simulink model "GreenCraneLagrangian"  (R2020b)
settings: Solver=FixedStepAuto  StartTime=0.0  StopTime=20  FixedStep=0.001  RelTol=1e-3  EnableMultiTasking=on
settings Model: Creator=dpadova  LastModifiedBy=hagen
settings SolverCC: AlgebraicLoopSolver=LineSearch
settings DataIOCC: LimitDataPoints=on  SaveFormat=Array  ReturnWorkspaceOutputs=off
settings OptimizationCC: ExpressionDepthLimit=2147483647  EfficientMapNaN2IntZero=off  LifeSpan=inf
settings DebuggingCC: AlgebraicLoopMsg=none  UnderspecifiedInitializationDetection=Classic  MergeDetectMultiDrivingBlocksExec=none  MaxConsecutiveZCsMsg=warning  StateNameClashWarn=warning  SFUnexpectedBacktrackingDiag=warning  SFNoUnconditionalDefaultTransitionDiag=warning  SFExecutionAtInitializationDiag=none  ArithmeticOperatorsInVariantConditions=warning
settings HardwareCC: ProdBitPerPointer=32  ProdBitPerSizeT=32  ProdBitPerPtrDiffT=32  ProdLargestAtomicFloat=None  ProdIntDivRoundTo=Undefined  ProdEndianess=Unspecified  ProdWordSize=32  ProdHWDeviceType=32-bit Generic  TargetBitPerPointer=64  TargetBitPerSizeT=64  TargetBitPerPtrDiffT=64  TargetLongLongMode=on  TargetIntDivRoundTo=Zero  TargetEndianess=LittleEndian  TargetWordSize=64  TargetHWDeviceType=MATLAB Host  ProdEqTarget=off
settings ModelReferenceCC: PropagateSignalLabelsOutOfModel=off
settings SFSimCC: SimUseLocalCustomCode=off  CustomCodeUndefinedFunction=UseInterfaceOnly
settings RTWCC: RTWUseLocalCustomCode=off
settings CodeAppCC: MaxIdLength=128
settings GRTTargetCC: TargetLangStandard=C89/C90 (ANSI)  CombineOutputUpdateFcns=off  GRTInterface=on
settings ConfigComp: CovMetricSettings=dw  CovSaveCumulativeToWorkspaceVar=on  CovSaveSingleToWorkspaceVar=on  CovExternalEMLEnable=off

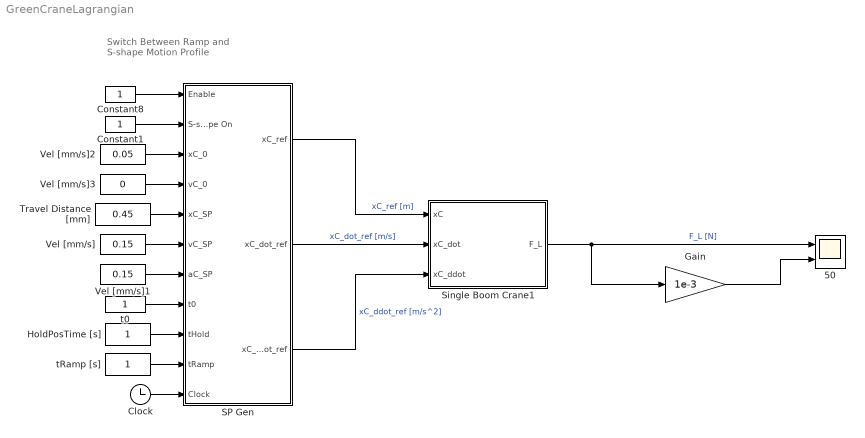
== system GreenCraneLagrangian ==
  note: Switch Between
      | Ramp and S-shape
      | Motion Profile
  50 : Scope  NumInputPorts=2
  Clock : Clock
  Constant1 : Constant  OutDataTypeStr=boolean
  Constant8 : Constant  OutDataTypeStr=boolean
  Gain : Gain  Gain=1e-3
  HoldPosTime [s] : Constant
  SP Gen : Subsystem
  Single Boom Crane1 : Subsystem
  Travel Distance [mm] : Constant  Value=0.45
  Vel [mm/s] : Constant  Value=0.15
  Vel [mm/s]1 : Constant  Value=0.15
  Vel [mm/s]2 : Constant  Value=0.05
  Vel [mm/s]3 : Constant  Value=0
  t0 : Constant
  tRamp [s] : Constant
  wires:
  Vel [mm/s]3/1 -> SP Gen/4(vC_0)
  t0/1 -> SP Gen/8(t0)
  HoldPosTime [s]/1 -> SP Gen/9(tHold)
  Clock/1 -> SP Gen/11(Clock)
  Travel Distance [mm]/1 -> SP Gen/5(xC_SP)
  Vel [mm/s]2/1 -> SP Gen/3(xC_0)
  Constant8/1 -> SP Gen/1(Enable)
  Vel [mm/s]/1 -> SP Gen/6(vC_SP)
  tRamp [s]/1 -> SP Gen/10(tRamp)
  Vel [mm/s]1/1 -> SP Gen/7(aC_SP)
  Constant1/1 -> SP Gen/2(S-shape On)
  SP Gen/1(xC_ref) -> Single Boom Crane1/1(xC)  "xC_ref [m]"
  SP Gen/2(xC_dot_ref) -> Single Boom Crane1/2(xC_dot)  "xC_dot_ref [m/s]"
  SP Gen/3("xC_ddot_ref ") -> Single Boom Crane1/3("xC_ddot ")  "xC_ddot_ref [m/s^2]"
  Single Boom Crane1/1(F_L) -> 50/1, Gain/1  "F_L [N]"
  Gain/1 -> 50/2

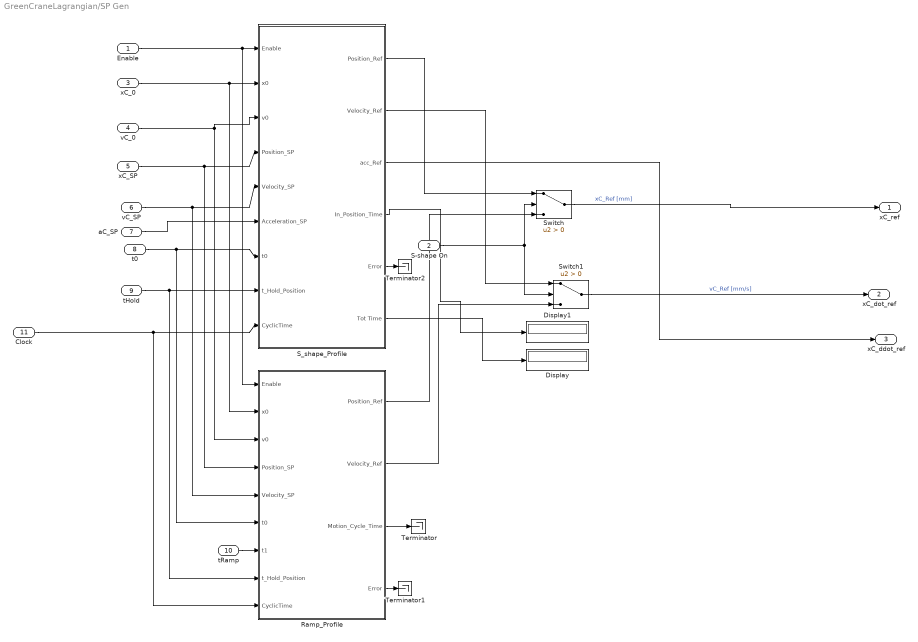
== system GreenCraneLagrangian/SP Gen ==
  Enable : Inport
  S-shape On : Inport  Port=2
  xC_0 : Inport  Port=3
  vC_0 : Inport  Port=4
  xC_SP : Inport  Port=5
  vC_SP : Inport  Port=6
  aC_SP : Inport  Port=7
  t0 : Inport  Port=8
  tHold : Inport  Port=9
  tRamp : Inport  Port=10
  Clock : Inport  Port=11
  Display : Display
  Display1 : Display
  Ramp_Profile : Subsystem  TreatAsAtomicUnit=on  VariantControl=Ramp_Profile
  S_shape_Profile : Subsystem  VariantControl=S_shape_Profile
  Switch : Switch  Criteria=u2 > Threshold
  Switch1 : Switch  Criteria=u2 > Threshold
  Terminator : Terminator
  Terminator1 : Terminator
  Terminator2 : Terminator
  xC_ref : Outport  VectorParamsAs1DForOutWhenUnconnected=off
  xC_dot_ref : Outport  Port=2  VectorParamsAs1DForOutWhenUnconnected=off
  "xC_ddot_ref " : Outport  Port=3  VectorParamsAs1DForOutWhenUnconnected=off
  wires:
  t0/1 -> Ramp_Profile/6(t0), S_shape_Profile/7(t0)
  vC_SP/1 -> Ramp_Profile/5(Velocity_SP), S_shape_Profile/5(Velocity_SP)
  xC_0/1 -> Ramp_Profile/2(x0), S_shape_Profile/2(x0)
  xC_SP/1 -> Ramp_Profile/4(Position_SP), S_shape_Profile/4(Position_SP)
  Enable/1 -> Ramp_Profile/1(Enable), S_shape_Profile/1(Enable)
  tHold/1 -> Ramp_Profile/8(t_Hold_Position), S_shape_Profile/8(t_Hold_Position)
  S_shape_Profile/1(Position_Ref) -> Switch/1
  Ramp_Profile/1(Position_Ref) -> Switch/3
  S_shape_Profile/2(Velocity_Ref) -> Switch1/1
  S-shape On/1 -> Switch/2, Switch1/2
  Ramp_Profile/2(Velocity_Ref) -> Switch1/3
  tRamp/1 -> Ramp_Profile/7(t1)
  S_shape_Profile/6(Tot Time) -> Display/1
  S_shape_Profile/4(" In_Position_Time") -> Display1/1
  vC_0/1 -> S_shape_Profile/3(v0), Ramp_Profile/3(v0)
  aC_SP/1 -> S_shape_Profile/6(Acceleration_SP)
  Clock/1 -> Ramp_Profile/9(CyclicTime), S_shape_Profile/9(CyclicTime)
  Switch/1 -> xC_ref/1  "xC_Ref [mm]"
  Switch1/1 -> xC_dot_ref/1  "vC_Ref [mm/s]"
  S_shape_Profile/3(acc_Ref) -> "xC_ddot_ref "/1
  Ramp_Profile/3(Motion_Cycle_Time) -> Terminator/1
  Ramp_Profile/4(Error) -> Terminator1/1
  S_shape_Profile/5(Error) -> Terminator2/1

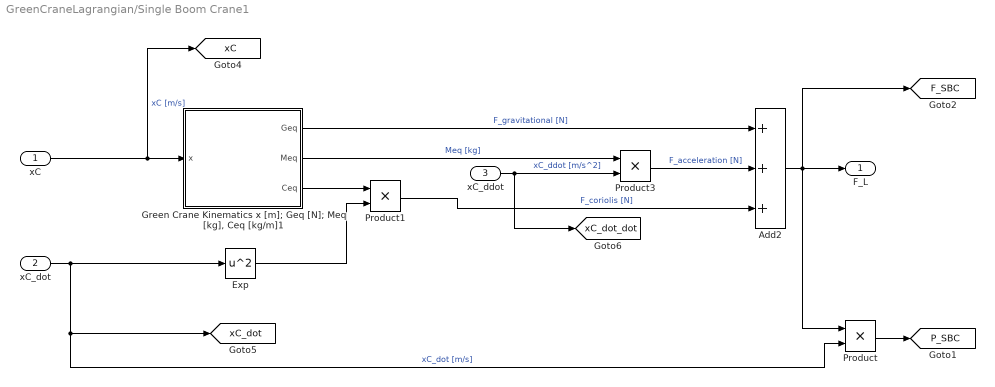
== system GreenCraneLagrangian/Single Boom Crane1 ==
  xC : Inport
  xC_dot : Inport  Port=2
  "xC_ddot " : Inport  Port=3
  Add2 : Sum  Inputs=+++
  Exp : Math  Operator=square  SaturateOnIntegerOverflow=on
  "Green Crane Kinematics x [m]; Geq [N]; Meq [kg], Ceq [kg/m]1" : MATLAB Function  TreatAsAtomicUnit=on
  Product : Product
  Product1 : Product
  Product3 : Product
  F_L : Outport
  tag scope: F_SBC=global, P_SBC=global, xC=global, xC_dot=global, xC_dot_dot=global
  wires:
  "Green Crane Kinematics x [m]; Geq [N]; Meq [kg], Ceq [kg/m]1"/2(Meq) -> Product3/1  "Meq [kg]"
  Add2/1 -> [F_SBC], Product/1, F_L/1
  "Green Crane Kinematics x [m]; Geq [N]; Meq [kg], Ceq [kg/m]1"/1(Geq) -> Add2/1  "F_gravitational [N]"
  Product3/1 -> Add2/2  "F_acceleration [N]"
  "Green Crane Kinematics x [m]; Geq [N]; Meq [kg], Ceq [kg/m]1"/3(Ceq) -> Product1/1
  Exp/1 -> Product1/2
  Product1/1 -> Add2/3  "F_coriolis [N]"
  "xC_ddot "/1 -> [xC_dot_dot], Product3/2  "xC_ddot [m/s^2]"
  xC_dot/1 -> Product/2, [xC_dot], Exp/1  "xC_dot [m/s]"
  xC/1 -> [xC], "Green Crane Kinematics x [m]; Geq [N]; Meq [kg], Ceq [kg/m]1"/1(x)  "xC [m/s]"
  Product/1 -> [P_SBC]

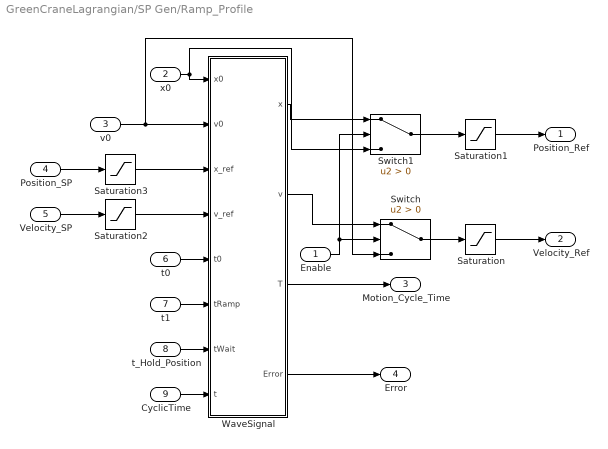
== system GreenCraneLagrangian/SP Gen/Ramp_Profile ==
  Enable : Inport  OutDataTypeStr=boolean
  x0 : Inport  Port=2
  v0 : Inport  Port=3
  Position_SP : Inport  Port=4
  Velocity_SP : Inport  Port=5
  t0 : Inport  Port=6
  t1 : Inport  Port=7
  t_Hold_Position : Inport  Port=8
  CyclicTime : Inport  Port=9
  Saturation : Saturate  UpperLimit=150  LowerLimit=-150
  Saturation1 : Saturate  UpperLimit=500  LowerLimit=0
  Saturation2 : Saturate  UpperLimit=150  LowerLimit=0
  Saturation3 : Saturate  UpperLimit=500  LowerLimit=0
  Switch : Switch  Criteria=u2 > Threshold
  Switch1 : Switch  Criteria=u2 > Threshold
  WaveSignal : MATLAB Function  TreatAsAtomicUnit=on
  Position_Ref : Outport  VectorParamsAs1DForOutWhenUnconnected=off
  Velocity_Ref : Outport  Port=2  VectorParamsAs1DForOutWhenUnconnected=off
  Motion_Cycle_Time : Outport  Port=3  VectorParamsAs1DForOutWhenUnconnected=off
  Error : Outport  Port=4  VectorParamsAs1DForOutWhenUnconnected=off
  wires:
  CyclicTime/1 -> WaveSignal/8(t)
  WaveSignal/2(v) -> Switch/1
  Switch/1 -> Saturation/1
  v0/1 -> Switch/3, WaveSignal/2(v0)
  t0/1 -> WaveSignal/5(t0)
  Position_SP/1 -> Saturation3/1
  t_Hold_Position/1 -> WaveSignal/7(tWait)
  Velocity_SP/1 -> Saturation2/1
  WaveSignal/1(x) -> Switch1/1
  WaveSignal/3(T) -> Motion_Cycle_Time/1
  Enable/1 -> Switch1/2, Switch/2
  x0/1 -> Switch1/3, WaveSignal/1(x0)
  Switch1/1 -> Saturation1/1
  Saturation/1 -> Velocity_Ref/1
  Saturation1/1 -> Position_Ref/1
  WaveSignal/4(Error) -> Error/1
  Saturation2/1 -> WaveSignal/4(v_ref)
  Saturation3/1 -> WaveSignal/3(x_ref)
  t1/1 -> WaveSignal/6(tRamp)

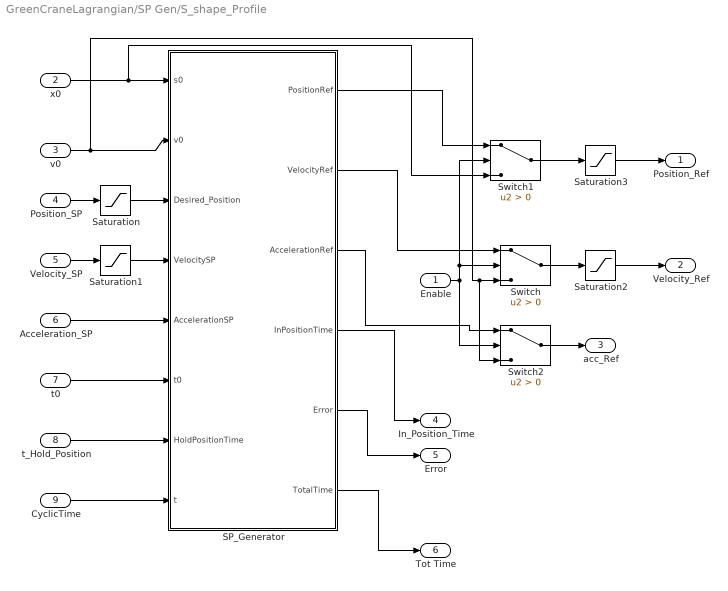
== system GreenCraneLagrangian/SP Gen/S_shape_Profile ==
  Enable : Inport  OutDataTypeStr=boolean
  x0 : Inport  Port=2
  v0 : Inport  Port=3
  Position_SP : Inport  Port=4
  Velocity_SP : Inport  Port=5
  Acceleration_SP : Inport  Port=6
  t0 : Inport  Port=7
  t_Hold_Position : Inport  Port=8
  CyclicTime : Inport  Port=9
  SP_Generator : MATLAB Function  TreatAsAtomicUnit=on
  Saturation : Saturate  UpperLimit=500  LowerLimit=0
  Saturation1 : Saturate  UpperLimit=150  LowerLimit=-150
  Saturation2 : Saturate  UpperLimit=150  LowerLimit=-150
  Saturation3 : Saturate  UpperLimit=500  LowerLimit=0
  Switch : Switch  Criteria=u2 > Threshold
  Switch1 : Switch  Criteria=u2 > Threshold
  Switch2 : Switch  Criteria=u2 > Threshold
  Position_Ref : Outport  VectorParamsAs1DForOutWhenUnconnected=off
  Velocity_Ref : Outport  Port=2  VectorParamsAs1DForOutWhenUnconnected=off
  acc_Ref : Outport  Port=3  VectorParamsAs1DForOutWhenUnconnected=off
  " In_Position_Time" : Outport  Port=4  VectorParamsAs1DForOutWhenUnconnected=off
  Error : Outport  Port=5  VectorParamsAs1DForOutWhenUnconnected=off
  Tot Time : Outport  Port=6  VectorParamsAs1DForOutWhenUnconnected=off
  wires:
  Saturation/1 -> SP_Generator/3(Desired_Position)
  Saturation1/1 -> SP_Generator/4(VelocitySP)
  t0/1 -> SP_Generator/6(t0)
  t_Hold_Position/1 -> SP_Generator/7(HoldPositionTime)
  Velocity_SP/1 -> Saturation1/1
  SP_Generator/4(InPositionTime) -> " In_Position_Time"/1
  CyclicTime/1 -> SP_Generator/8(t)
  SP_Generator/5(Error) -> Error/1
  Position_SP/1 -> Saturation/1
  Saturation2/1 -> Velocity_Ref/1
  Switch/1 -> Saturation2/1
  x0/1 -> Switch1/3, SP_Generator/1(s0)
  SP_Generator/1(PositionRef) -> Switch1/1
  Saturation3/1 -> Position_Ref/1
  Enable/1 -> Switch2/2, Switch1/2, Switch/2
  SP_Generator/2(VelocityRef) -> Switch/1
  Switch1/1 -> Saturation3/1
  SP_Generator/6(TotalTime) -> Tot Time/1
  Acceleration_SP/1 -> SP_Generator/5(AccelerationSP)
  v0/1 -> Switch2/3, Switch/3, SP_Generator/2(v0)
  SP_Generator/3(AccelerationRef) -> Switch2/1
  Switch2/1 -> acc_Ref/1

== matlab function GreenCraneLagrangian/Single Boom Crane1/Green Crane Kinematics x [m]; Geq [N]; Meq [kg], Ceq [kg//m]1 ==
  data: x input; Geq output; Meq output; Ceq output

function [Geq, Meq, Ceq]  = fcn(x)

% Mechanical Model Green Crane @ UiA Laboratory 

% Parameters 
L_AGx = 3139/1000;            % [m]
L_AGy = 64*(1/1000);          % [m]
L_ACx = 550*(1/1000);         % [m]
L_ACy = 130*(1/1000);         % [m]
L_ABx = 420*(1/1000);         % [m]
L_ABy = 1055*(1/1000);        % [m]
L_AB = sqrt(L_ABx^2+L_ABy^2); % [m]
L_AC = sqrt(L_ACx^2+L_ACy^2); % [m]
L_AG = sqrt(L_AGx^2+L_AGy^2); % [m]
m_cm = 415.075;               % [kg]
J_A = 4251.2;                 % [kg*m^2]
J_cm = J_A-L_AG^2*m_cm;       % [kg*m^2]
L_min = 772*(1/1000);         % [m]
g = 9.82;                     % [m/s^2]

% Gravitational Load [N]
Geq = -0.2e1*sqrt(-(x-L_AB+L_min+L_AC)*(x+L_min-L_AC-L_AB)*(x+L_AB+L_min-L_AC)*(x+L_AB+L_min+L_AC))*g*m_cm*(cos(acos((L_AB^2+L_AC^2-(x+L_min)^2)/L_AC/L_AB/0.2e1)-atan(L_ABy/L_ABx)+atan(L_ACy/L_ACx)+atan(L_AGy/L_AGx))*L_AGx-sin(acos((L_AB^2+L_AC^2-(x+L_min)^2)/L_AC/L_AB/0.2e1)-atan(L_ABy/L_ABx)+atan(L_ACy/L_ACx)+atan(L_AGy/L_AGx))*L_AGy)*(x+L_min)/(x-L_AB+L_min+L_AC)/(x+L_min-L_AC-L_AB)/(x+L_AB+L_min-L_AC)/(x+L_AB+L_min+L_AC);

% Equalent Inertial Load [kg]
Meq = -4*(L_AGx^2*(x+L_min)*m_cm+L_AGy^2*(x+L_min)*m_cm+(x+L_min)*J_cm)*(x+L_min)/(-x+L_AB-L_min-L_AC)/(-x+L_AB-L_min+L_AC)/(x+L_AB+L_min+L_AC)/(x+L_AB+L_min-L_AC);

% Coriolis Force [N/(m/s)^2] = [kg/m]
Ceq = 4*((L_AGx^2+L_AGy^2)*m_cm+J_cm)*(x+L_min)*(-L_AB^2+L_AC^2+(x+L_min)^2)*(L_AB^2-L_AC^2+(x+L_min)^2)/(x+L_min-L_AC-L_AB)^2/(x-L_AB+L_min+L_AC)^2/(x+L_AB+L_min+L_AC)^2/(x+L_AB+L_min-L_AC)^2;

== matlab function GreenCraneLagrangian/SP Gen/S_shape_Profile/SP_Generator ==
  data: PositionRef output; VelocityRef output; AccelerationRef output; InPositionTime output; s0 input; v0 input; Desired_Position input; VelocitySP input; AccelerationSP input; t0 input; HoldPositionTime input; t input; Error output; TotalTime output
function [PositionRef,VelocityRef,AccelerationRef, InPositionTime, Error, TotalTime] = fcn(s0,v0, Desired_Position,VelocitySP, AccelerationSP, t0,HoldPositionTime,t)


PositionSP = Desired_Position - s0;

a0 = 0;
j0 = 0;


vel=VelocitySP;
as=AccelerationSP;
% Input velocity 
vs=vel; %[rad/s]
% Delta velocity 
dv=(vs-v0); %[rad/s]     
% Max Jerk Considerations
jm=as^2/dv; %%[rad/s^3] 
% Constant Velocity periodes
s_acc=(vs^2-v0^2)/as;
CstVelTime=(PositionSP-2*s_acc)/vs;
if CstVelTime < 0
Error = 1;
else 
Error = 0;
end

% Time periodes,
t1=t0+(as/jm);
t2=t1+(as/jm);
t3=t2+CstVelTime;
t4=t3+(as/jm);
t5=t4+(as/jm);
t6=t5+HoldPositionTime;
t7=t6+(as/jm);
t8=t7+(as/jm);
t9=t8+CstVelTime;
t10=t9+(as/jm);
t11=t10+(as/jm);
% Position and Velocity Constants
sh=(v0+(as^2)/(6*jm))*(as/jm);
vh=(vs-v0)/2;
s3=s_acc+vs*(t3-t2);
s4=s3+vs*(t4-t3)-jm*((t4-t3)^3)/6;
v4=vs-jm*((t4-t3)^2)/2;
s5=s0+jm*((t5-t4)^3)/6-as*((t5-t4)^2)/2+v4*(t5-t4)+s4;
%s6=s5+(s0+v0*(t7-t6)+jm*((t7-t6)^3)/6);
s7= s5-(s_acc+vs*(t9-t8));
s8= s7-(vs*(t10-t9)-jm*((t10-t9)^3)/6);
%s9= s8-(jm*((t11-t10)^3)/6-as*((t11-t10)^2)/2+v4*(t11-t10));
%Phase0
if  Error == 1   
s = s0;
v = v0;
a = a0;
j=j0; 
elseif  (t >= 0) && (t <= t0)    
s = s0;
v = v0;
a = a0;
j=j0;        
%Phase1 - concave Acc
elseif  (t >= t0) && (t <= (t1))
s = s0+v0*(t-t0)+jm*((t-t0)^3)/6;
v = v0+jm*((t-t0)^2)/2;
a = jm*(t-t0);
j=jm;
%Phase2 - convex Acc
elseif (t >= (t1)) && (t <= (t2))
s = s0+sh+vh*(t-t1)+as*((t-t1)^2)/2-jm*((t-t1)^3)/6;
v = vh+as*(t-t1)-jm*((t-t1)^2)/2;
a = as-jm*(t-t1);
j = -jm; 
%Phase3 - constant velocity
elseif (t >= t2) && (t <= t3)
s = s0+s_acc+vs*(t-t2);
v = vs;
a = 0;
j = 0;   
%Phase4 - convex Dec
elseif (t >= t3) && (t <= t4)
s = s0+s3+vs*(t-t3)-jm*((t-t3)^3)/6;
v = vs-jm*((t-t3)^2)/2;
a = -jm*(t-t3);
j = -jm; 
%Phase5 - concav Dec
elseif (t >= t4) && (t <= t5)
s = s0+jm*((t-t4)^3)/6-as*((t-t4)^2)/2+v4*(t-t4)+s4;
v = jm*((t-t4)^2)/2-as*(t-t4)+v4;
a = jm*(t-t4)-as;
j=jm; 
%Phase6 - holding position
elseif (t >= t5) && (t <= t6)
s = s5;
v = 0;
a = 0;
j = 0;  
%Phase7 - concave Dec
elseif (t >= t6) && (t <= t7)
s = s5-(v0*(t-t6)+jm*((t-t6)^3)/6);
v = -(v0+jm*((t-t6)^2)/2);
a = -jm*(t-t6);
j=-jm;
%Phase8 - convex Dec
elseif (t >= t7) && (t <= t8)    
s = s5-(sh+vh*(t-t7)+as*((t-t7)^2)/2-jm*((t-t7)^3)/6);
v = -(vh+as*(t-t7)-jm*((t-t7)^2)/2);
a = -(as-jm*(t-t7));
j = jm; 
%Phase9 - constant velocity
elseif (t >= t8) && (t <= t9)
s = s5-(s_acc+vs*(t-t8));
v = -vs;
a = 0;
j = 0;     
%Phase10 - concav Acc
elseif (t >= t9) && (t <= t10)
s = s7-(vs*(t-t9)-jm*((t-t9)^3)/6);
v = -(vs-jm*((t-t9)^2)/2);
a = jm*(t-t9);
j = jm; 
%Phase11 - convex Acc
elseif (t >= t10) && (t <= t11)
s = s8-(jm*((t-t10)^3)/6-as*((t-t10)^2)/2+v4*(t-t10));
v = -(jm*((t-t10)^2)/2-as*(t-t10)+v4);
a = -(jm*(t-t10)-as);
j=-jm; 
%Phase12 - hold position
else
s = s0;
v = v0;
a = a0;
j = j0;
end

if t == 0
PositionRef=s0; %[mm]
else 
PositionRef=s; %[mm]
end 

InPositionTime=t5; %[s]
TotalTime=t11; 
VelocityRef=v; %[mm/s]
AccelerationRef=a; %[mm/s^2]
JerkRef=j; % %[mm/s^3]

== matlab function GreenCraneLagrangian/SP Gen/Ramp_Profile/WaveSignal ==
  data: x0 input; v0 input; x_ref input; x output; v_ref input; t0 input; tRamp input; tWait input; v output; t input; T output; Error output
function [x,v,T, Error] = fcn(x0,v0, x_ref,v_ref,t0,tRamp,tWait,t)
x_SP = x_ref - x0;
vs=v_ref;
slopeExt=v0-vs;
slopeRetr=-vs-v0;

as = vs/tRamp;
s_acc=(vs^2-v0^2)/as;

tHold=(x_SP-s_acc)/vs;

if tHold < 0 
Error = 1;
else 
Error = 0;
end

t1=tRamp;
t2=tHold; 
t3=tRamp;
t4=tWait;
t5=t1;
t6=t2;
t7=t3;

x = x0;
x1 = x0 + v0*((t0+t1)-t0)-(slopeExt/t1)*((t0+t1)-t0)^2/2;
x2 = x1 + vs*((t0+t1+t2)-(t0+t1)); 
x4 = x_ref - v0*((t0+t1+t2+t3+t4+t5)-(t0+t1+t2+t3+t4))+(slopeRetr/t5)*((t0+t1+t2+t3+t4+t5)-(t0+t1+t2+t3+t4))^2/2; 
x5 = x4-vs*((t0+t1+t2+t3+t4+t5+t6)-(t0+t1+t2+t3+t4+t5));  

if Error == 1
x = x0;
v = v0; 
elseif t>=0 && t<t0
x = x0; 
v = v0;
elseif t>=t0 && t<(t0+t1)
x = x0 + v0*(t-t0)-(slopeExt/t1)*(t-t0)^2/2;
v = v0-(slopeExt/t1)*(t-t0);  
elseif t>=(t0+t1) && t<(t0+t1+t2)
x = x1 + vs*(t-(t0+t1)); 
v = vs; 
elseif t>=(t0+t1+t2) && t<(t0+t1+t2+t3)
x = x2+vs*(t-(t0+t1+t2))+(slopeExt/t3)*(t-(t0+t1+t2))^2/2; 
v = vs+(slopeExt/t3)*(t-(t0+t1+t2));   
elseif t>=(t0+t1+t2+t3) && t<(t0+t1+t2+t3+t4)
x = x_ref;
v = v0;  
elseif t>=(t0+t1+t2+t3+t4) && t<(t0+t1+t2+t3+t4+t5)
x = x_ref - v0*(t-(t0+t1+t2+t3+t4))+(slopeRetr/t5)*(t-(t0+t1+t2+t3+t4))^2/2; 
v = v0+(slopeRetr/t5)*(t-(t0+t1+t2+t3+t4));     
elseif t>=(t0+t1+t2+t3+t4+t5) && t<(t0+t1+t2+t3+t4+t5+t6)
x = x4-vs*(t-(t0+t1+t2+t3+t4+t5));   
v = -vs;    
elseif t>=(t0+t1+t2+t3+t4+t5+t6) && t<(t0+t1+t2+t3+t4+t5+t6+t7)
x = x5-vs*(t-(t0+t1+t2+t3+t4+t5+t6))-(slopeRetr/t3)*(t-(t0+t1+t2+t3+t4+t5+t6))^2/2;    
v = -vs-(slopeRetr/t3)*(t-(t0+t1+t2+t3+t4+t5+t6));     
else 
x = x0;
v = v0; 
end

T = t0+t1+t2+t3+t4+t5+t6+t7;
